simulink model "f2"  (R2015b)
settings: Solver=VariableStepAuto  StartTime=0.0  StopTime=1e-5  RelTol=1e-3
libraries: simulink_extras x2, commchan3 x1, dsparch4 x1, commrflib2 x1, commsynccomp2 x1, dspsigops x1
settings Model: Creator=dimple  LastModifiedBy=dimple

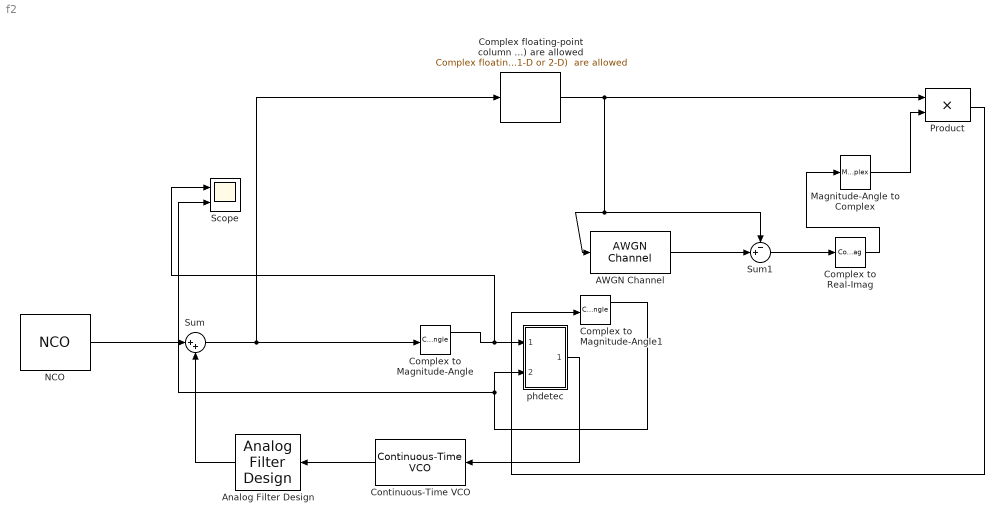
== system f2 ==
  AWGN Channel : commchan3/AWGN Channel  InputProcessing=Columns as channels (frame based)  seed=2537  noiseMode=Variance from mask  EbNodB=10  EsNodB=10  SNRdB=0  bitsPerSym=1  Ps=1  Tsym=1  variance=2
  Analog Filter Design : dsparch4/Analog Filter Design  method=Butterworth  filttype=Lowpass  N=5  Wlo=1e6*2*pi  Whi=80  Rp=2  Rs=40
  Complex floating-point column vectors (1-D or 2-D) are allowed : commrflib2/Phase Noise/Complex floating-point  column vectors (1-D or 2-D)  are allowed
  Complex to Magnitude-Angle : ComplexToMagnitudeAngle
  Complex to Magnitude-Angle1 : ComplexToMagnitudeAngle
  Complex to Real-Imag : ComplexToRealImag  Output=Real
  Continuous-Time VCO : commsynccomp2/Continuous-Time VCO  Ac=1  Fc=1e6  Kc=1e5  Ph=0
  Magnitude-Angle to Complex : MagnitudeAngleToComplex  Input=Angle  ConstantPart=1
  NCO : dspsigops/NCO  AccIncSrc=Specify via dialog  AccInc=100  PhaseOffsetSrc=Specify via dialog  PhaseOffset=0  AccumWL=16  HasDither=on  DitherWL=4  PNgeneratorLength=19  HasPhaseQuantizer=on  TableDepth=12  HasOutputPhaseError=off  Formula=Complex exponential  DataType=double  OutputWL=16  OutputFL=14  CompMethod=Table lookup (no interpolation)  SampleTime=1  SamplesPerFrame=1  OutputFrames=off
  Product : Product  SaturateOnIntegerOverflow=on  InputSameDT=on  OutDataTypeStr=Inherit: Same as first input
  Scope : Scope  NumInputPorts=2
  Sum : Sum  Inputs=|++
  Sum1 : Sum  Inputs=-+|  SaturateOnIntegerOverflow=on  InputSameDT=on  OutDataTypeStr=Inherit: Same as first input
  "phdetec " : Subsystem
  wires:
  NCO/1 -> Sum/1
  Sum/1 -> Complex floating-point column vectors (1-D or 2-D) are allowed/1, Complex to Magnitude-Angle/1
  Continuous-Time VCO/1 -> Analog Filter Design/1
  Analog Filter Design/1 -> Sum/2
  Complex to Magnitude-Angle/1 -> Scope/1, "phdetec "/1(In1)
  "phdetec "/1("Out ") -> Continuous-Time VCO/1
  Complex to Magnitude-Angle1/1 -> Scope/2, "phdetec "/2(In2)
  Magnitude-Angle to Complex/1 -> Product/2
  Complex floating-point column vectors (1-D or 2-D) are allowed/1 -> AWGN Channel/1, Sum1/1, Product/1
  AWGN Channel/1 -> Sum1/2
  Sum1/1 -> Complex to Real-Imag/1
  Complex to Real-Imag/1 -> Magnitude-Angle to Complex/1
  Product/1 -> Complex to Magnitude-Angle1/1

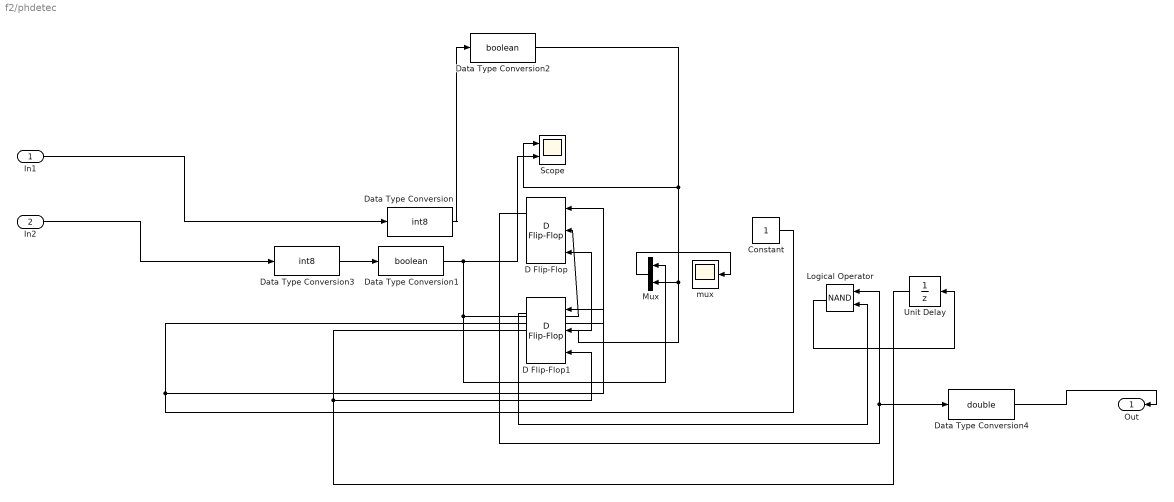
== system f2/phdetec  ==
  In1 : Inport
  In2 : Inport  Port=2
  Constant : Constant  OutDataTypeStr=boolean
  D Flip-Flop : simulink_extras/Flip Flops/D Flip-Flop
  D Flip-Flop1 : simulink_extras/Flip Flops/D Flip-Flop
  Data Type Conversion : DataTypeConversion  OutDataTypeStr=int8
  Data Type Conversion1 : DataTypeConversion  OutDataTypeStr=boolean
  Data Type Conversion2 : DataTypeConversion  OutDataTypeStr=boolean
  Data Type Conversion3 : DataTypeConversion  OutDataTypeStr=int8
  Data Type Conversion4 : DataTypeConversion  OutDataTypeStr=double
  Logical Operator : Logic  Operator=NAND  AllPortsSameDT=off  OutDataTypeStr=boolean
  Mux : Mux  Inputs=2
  Scope : Scope  NumInputPorts=2
  Unit Delay : UnitDelay  SampleTime=0.01
  "mux " : Scope
  "Out " : Outport
  wires:
  Data Type Conversion1/1 -> D Flip-Flop/2, Mux/1, Scope/2
  D Flip-Flop1/1 -> Logical Operator/2
  D Flip-Flop/1 -> Logical Operator/1, Data Type Conversion4/1
  In2/1 -> Data Type Conversion3/1
  Constant/1 -> D Flip-Flop/1, D Flip-Flop1/1
  Mux/1 -> "mux "/1
  Logical Operator/1 -> Unit Delay/1
  Unit Delay/1 -> D Flip-Flop/3, D Flip-Flop1/3
  Data Type Conversion2/1 -> Scope/1, D Flip-Flop1/2, Mux/2
  Data Type Conversion3/1 -> Data Type Conversion1/1
  In1/1 -> Data Type Conversion/1
  Data Type Conversion/1 -> Data Type Conversion2/1
  Data Type Conversion4/1 -> "Out "/1
